simulink model "unitdelay"  (Simulink 6.6)
settings: Solver=FixedStepDiscrete  StartTime=0.0  StopTime=10.0  FixedStep=1  RelTol=1e-3
settings Model: Creator=ksmyth  LastModifiedBy=ksmyth

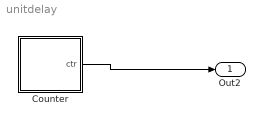
== system unitdelay ==
  Counter : Stateflow chart
  Out2 : Outport
  wires:
  Counter/1(ctr) -> Out2/1

== stateflow chart Counter ==
  state s1
  (default) -> s1
  s1 -> s1 [order 1] : [ctr < 4] / ctr = ctr+1;
  s1 -> s1 [order 2] : [ctr >= 4] / ctr = 0;
  data: ctr output double =1
